simulink model "Mov_theta"  (R2017a)
settings: Solver=VariableStepAuto  StartTime=0.0  StopTime=15  RelTol=1e-3
settings Model: Creator=13199959938  LastModifiedBy=13199959938

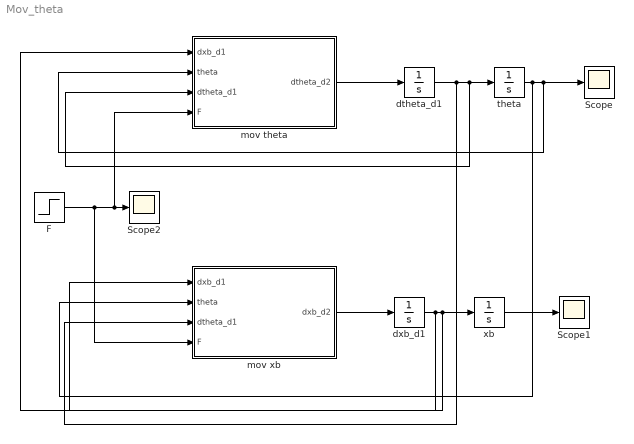
== system Mov_theta ==
  F : Step  Time=4  After=540  SampleTime=0
  Scope : Scope
  Scope1 : Scope
  Scope2 : Scope
  dtheta_d1 : Integrator
  dxb_d1 : Integrator
  mov theta : MATLAB Function  TreatAsAtomicUnit=on
  mov xb : MATLAB Function  TreatAsAtomicUnit=on
  theta : Integrator
  xb : Integrator
  wires:
  mov xb/1(dxb_d2) -> dxb_d1/1
  mov theta/1(dtheta_d2) -> dtheta_d1/1
  dtheta_d1/1 -> mov xb/3(dtheta_d1), mov theta/3(dtheta_d1), theta/1
  theta/1 -> mov xb/2(theta), mov theta/2(theta), Scope/1
  dxb_d1/1 -> mov xb/1(dxb_d1), mov theta/1(dxb_d1), xb/1
  xb/1 -> Scope1/1
  F/1 -> mov xb/4(F), mov theta/4(F), Scope2/1

== matlab function Mov_theta/mov xb ==
  data: dxb_d1 input; dxb_d2 output; theta input; dtheta_d1 input; F input
function dxb_d2 = mov_xb(dxb_d1, theta, dtheta_d1, F)
    g = 9.81; % m/s^2
    l = 1.30; % m
    m = 120; % kg
    M = 54; % kg
    b = 1.3; % atrito viscoso com o ar
    d = 97.2; % Ns/M
    
    dxb_d2 = (F-d*dxb_d1-m*l*sin(theta)*dtheta_d1^2+m*g*sin(theta)*cos(theta)-(b*dtheta_d1*cos(theta))/l)/((M+m*(sin(theta))^2));

== matlab function Mov_theta/mov theta ==
  data: dxb_d1 input; dtheta_d2 output; theta input; dtheta_d1 input; F input
function dtheta_d2 = mov_theta(dxb_d1, theta, dtheta_d1, F)
    g = 9.81; % m/s^2
    l = 1.30; % m
    m = 120; % kg
    M = 54; % kg
    b = 1.3; % atrito viscoso com o ar
    d = 97.2; % Ns/M
    
    dtheta_d2 = ((M+m)*g*l*sin(theta)+l*cos(theta)*(F-d*dxb_d1-m*l*sin(theta)*dtheta_d1^2)-((M+m)*b*dtheta_d1)/m)/(l^2*(M+m*(sin(theta))^2));
